simulink model "switching_controller_nominal"  (R2022a)
settings: Solver=VariableStepAuto  StartTime=0.0  StopTime=10.0  RelTol=1e-3
model workspace (MAT data in the model file):
  PID_TRESH = 0.3
undefined symbols (not defined in the file or in its folder): DiscIntNeverNeededParam
libraries: simulink x1
settings Model: LastModifiedBy=alex
settings OptimizationCC: BlockReduction=off  BooleanDataType=off
settings DebuggingCC: SaveWithParameterizedLinksMsg=none  UnderspecifiedInitializationDetection=Classic  MergeDetectMultiDrivingBlocksExec=none  SignalResolutionControl=TryResolveAllWithWarning
settings HardwareCC: TargetUnknown=on
settings ModelReferenceCC: PropagateSignalLabelsOutOfModel=off

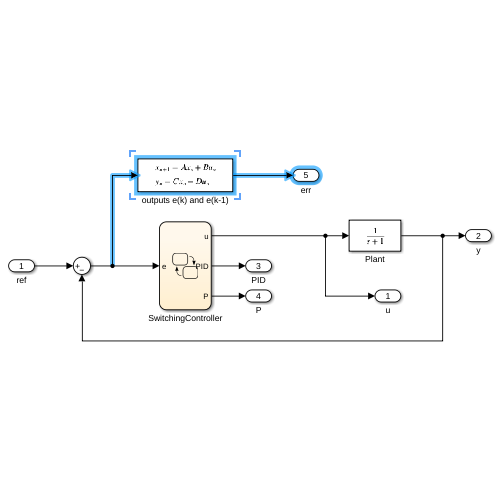
[thumbnail: Simulink's stored preview of the top-level diagram]
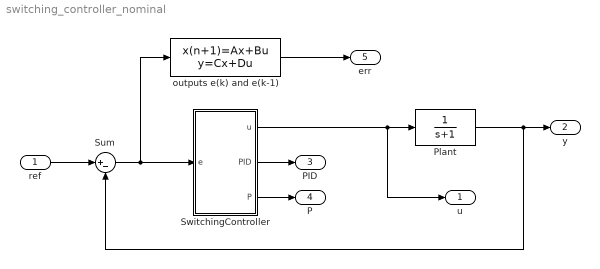
== system switching_controller_nominal ==
  ref : Inport
  Plant : TransferFcn  Denominator=[1 1]
  Sum : Sum  Inputs=|+-
  SwitchingController : Stateflow chart  TreatAsAtomicUnit=on
  outputs e(k) and e(k-1) : DiscreteStateSpace  A=[0 0; 1 0]  B=[1 ; 0]  C=[0 0; 1 0]  D=[1 ; 0]  SampleTime=-1
  u : Outport
  y : Outport  Port=2
  PID : Outport  Port=3
  P : Outport  Port=4
  err : Outport  Port=5
  wires:
  Sum/1 -> outputs e(k) and e(k-1)/1, SwitchingController/1(e)
  SwitchingController/2(" PID") -> PID/1
  SwitchingController/3(" P") -> P/1
  SwitchingController/1(u) -> Plant/1, u/1
  Plant/1 -> Sum/2, y/1
  ref/1 -> Sum/1
  outputs e(k) and e(k-1)/1 -> err/1

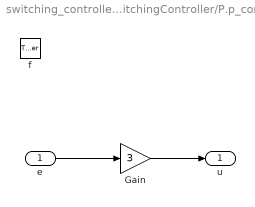
== system switching_controller_nominal/SwitchingController/P.p_control ==
  e : Inport
  f : TriggerPort  TriggerType=function-call  VariantControl=(inherit)
      settings: CopyFcn=Stateflow.SLINSF.SimulinkMan.removeBlockPreDeleteFcn  PreDeleteFcn=Stateflow.SLINSF.SimulinkMan.unsafePredeleteFcn
  Gain : Gain  Gain=3
  u : Outport  VectorParamsAs1DForOutWhenUnconnected=off
  wires:
  e/1 -> Gain/1
  Gain/1 -> u/1

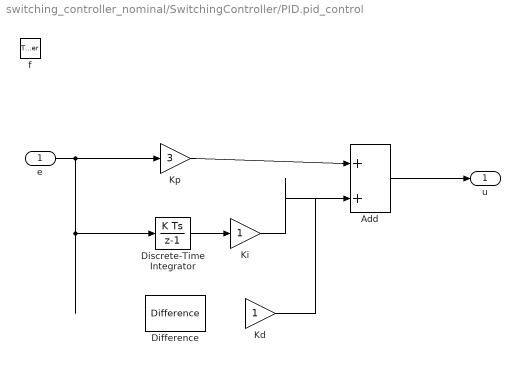
== system switching_controller_nominal/SwitchingController/PID.pid_control ==
  e : Inport
  f : TriggerPort  TriggerType=function-call  VariantControl=(inherit)
      settings: CopyFcn=Stateflow.SLINSF.SimulinkMan.removeBlockPreDeleteFcn  PreDeleteFcn=Stateflow.SLINSF.SimulinkMan.unsafePredeleteFcn
  Add : Sum  Inputs=+++
  Difference : simulink/Discrete/Difference  ICPrevInput=0.0  OutMin=[]  OutMax=[]  OutDataType=fixdt(1, 16)  OutScaling=2^-10  DoSatur=off
  Discrete-Time Integrator : DiscreteIntegrator  SampleTime=-1  ICPrevOutput=DiscIntNeverNeededParam  ICPrevScaledInput=DiscIntNeverNeededParam
  Kd : Gain
  Ki : Gain
  Kp : Gain  Gain=3
  u : Outport  VectorParamsAs1DForOutWhenUnconnected=off
  wires:
  e/1 -> Kp/1, Discrete-Time Integrator/1
  Kp/1 -> Add/1
  Add/1 -> u/1
  Discrete-Time Integrator/1 -> Ki/1
  ? -> Kd/1
  Ki/1 -> Add/2
  Kd/1 -> ?

== stateflow chart switching_controller_nominal/SwitchingController ==
  state STEADY
    entry: u = 0;
  state P
    du:
    u = p_control(e);
    state u = p_control(e) [function]
  state PID
    du:
    u = pid_control(e);
    state u = pid_control(e) [function]
  (default) -> STEADY
  STEADY -> P : [e > -0.01]
  P -> PID : [e < PID_TRESH]
  data: e function_input; u function_output; e function_input; u function_output; e input; u output double; PID output boolean; PID_TRESH parameter; P output boolean
